simulink model "test_mdl_NI"  (R2018a)
settings: Solver=VariableStepAuto  StartTime=0.0  StopTime=10.0  RelTol=1e-3
(part 5 of 24)

== system test_mdl_NI/CAN_Signal/BCM/PaakRqData1_0x468 ==
  in : Inport
  KeyPadCodeProg_D_Stat : Subsystem
  PaakTrgtData_D_Rq : Subsystem
  PaakTrgtPssvData_No_Rq : Subsystem
  PaakTrgtRollCode_No_Rq : Subsystem
  PaakTrgtType_D_Rq : Subsystem
  PaakTrgtZone_D_Rq : Subsystem
  bus_creator : BusCreator  Inputs=6
  bus_selector : BusSelector  OutputSignals=PaakTrgtPssvData_No_Rq,PaakTrgtData_D_Rq,PaakTrgtRollCode_No_Rq,PaakTrgtType_D_Rq,PaakTrgtZone_D_Rq,KeyPadCodeProg_D_Stat
  out_port : Outport
  wires:
  bus_creator/1 -> out_port/1  "PaakRqData1_0x468"
  PaakTrgtPssvData_No_Rq/1(out) -> bus_creator/1  "PaakTrgtPssvData_No_Rq"
  PaakTrgtData_D_Rq/1(out) -> bus_creator/2  "PaakTrgtData_D_Rq"
  PaakTrgtRollCode_No_Rq/1(out) -> bus_creator/3  "PaakTrgtRollCode_No_Rq"
  PaakTrgtType_D_Rq/1(out) -> bus_creator/4  "PaakTrgtType_D_Rq"
  PaakTrgtZone_D_Rq/1(out) -> bus_creator/5  "PaakTrgtZone_D_Rq"
  KeyPadCodeProg_D_Stat/1(out) -> bus_creator/6  "KeyPadCodeProg_D_Stat"
  bus_selector/1 -> PaakTrgtPssvData_No_Rq/1(in)  "<PaakTrgtPssvData_No_Rq>"
  bus_selector/2 -> PaakTrgtData_D_Rq/1(in)  "<PaakTrgtData_D_Rq>"
  bus_selector/3 -> PaakTrgtRollCode_No_Rq/1(in)  "<PaakTrgtRollCode_No_Rq>"
  bus_selector/4 -> PaakTrgtType_D_Rq/1(in)  "<PaakTrgtType_D_Rq>"
  bus_selector/5 -> PaakTrgtZone_D_Rq/1(in)  "<PaakTrgtZone_D_Rq>"
  bus_selector/6 -> KeyPadCodeProg_D_Stat/1(in)  "<KeyPadCodeProg_D_Stat>"
  in/1 -> bus_selector/1

== system test_mdl_NI/CAN_Signal/BCM/PaakRqData2_0x469 ==
  in : Inport
  PaakTrgtActvData_No_Rq : Subsystem
  bus_creator : BusCreator  Inputs=1
  bus_selector : BusSelector  OutputSignals=PaakTrgtActvData_No_Rq
  out_port : Outport
  wires:
  bus_creator/1 -> out_port/1  "PaakRqData2_0x469"
  PaakTrgtActvData_No_Rq/1(out) -> bus_creator/1  "PaakTrgtActvData_No_Rq"
  bus_selector/1 -> PaakTrgtActvData_No_Rq/1(in)  "<PaakTrgtActvData_No_Rq>"
  in/1 -> bus_selector/1

== system test_mdl_NI/CAN_Signal/BCM/Personality_BCM2_Data_0x3EB ==
  in : Inport
  AssocConfirm_D_Actl : Subsystem
  EmPrflKeyAssoc_D_Stat : Subsystem
  EmPrflNo_D_Stat : Subsystem
  Pers1Key_D_Stat : Subsystem
  Pers2Key_D_Stat : Subsystem
  Pers3Key_D_Stat : Subsystem
  Pers4Key_D_Stat : Subsystem
  PersConflict_D_Actl : Subsystem
  PersNoPos_D_Actl : Subsystem
  PersNo_D_Actl : Subsystem
  PersRecallSrc_D_Actl : Subsystem
  PersSetupAccessCtrl : Subsystem
  PersSetupRestr_D_Actl : Subsystem
  PersSetup_No_Actl : Subsystem
  RecallEvent_No_Cnt : Subsystem
  VehKeyActv_D_Stat : Subsystem
  bus_creator : BusCreator  Inputs=16
  bus_selector : BusSelector  OutputSignals=RecallEvent_No_Cnt,AssocConfirm_D_Actl,Pers1Key_D_Stat,PersNo_D_Actl,PersConflict_D_Actl,PersSetupRestr_D_Actl,PersSetupAccessCtrl,PersNoPos_D_Actl,PersSetup_No_Actl,VehKeyActv_D_Stat,Pers2Key_D_Stat,Pers3Key_D_Stat,EmPrflKeyAssoc_D_Stat,EmPrflNo_D_Stat,Pers4Key_D_Stat,PersRecallSrc_D_Actl
  out_port : Outport
  wires:
  bus_creator/1 -> out_port/1  "Personality_BCM2_Data_0x3EB"
  RecallEvent_No_Cnt/1(out) -> bus_creator/1  "RecallEvent_No_Cnt"
  AssocConfirm_D_Actl/1(out) -> bus_creator/2  "AssocConfirm_D_Actl"
  Pers1Key_D_Stat/1(out) -> bus_creator/3  "Pers1Key_D_Stat"
  PersNo_D_Actl/1(out) -> bus_creator/4  "PersNo_D_Actl"
  PersConflict_D_Actl/1(out) -> bus_creator/5  "PersConflict_D_Actl"
  PersSetupRestr_D_Actl/1(out) -> bus_creator/6  "PersSetupRestr_D_Actl"
  PersSetupAccessCtrl/1(out) -> bus_creator/7  "PersSetupAccessCtrl"
  PersNoPos_D_Actl/1(out) -> bus_creator/8  "PersNoPos_D_Actl"
  PersSetup_No_Actl/1(out) -> bus_creator/9  "PersSetup_No_Actl"
  VehKeyActv_D_Stat/1(out) -> bus_creator/10  "VehKeyActv_D_Stat"
  Pers2Key_D_Stat/1(out) -> bus_creator/11  "Pers2Key_D_Stat"
  Pers3Key_D_Stat/1(out) -> bus_creator/12  "Pers3Key_D_Stat"
  EmPrflKeyAssoc_D_Stat/1(out) -> bus_creator/13  "EmPrflKeyAssoc_D_Stat"
  EmPrflNo_D_Stat/1(out) -> bus_creator/14  "EmPrflNo_D_Stat"
  Pers4Key_D_Stat/1(out) -> bus_creator/15  "Pers4Key_D_Stat"
  PersRecallSrc_D_Actl/1(out) -> bus_creator/16  "PersRecallSrc_D_Actl"
  bus_selector/1 -> RecallEvent_No_Cnt/1(in)  "<RecallEvent_No_Cnt>"
  bus_selector/2 -> AssocConfirm_D_Actl/1(in)  "<AssocConfirm_D_Actl>"
  bus_selector/3 -> Pers1Key_D_Stat/1(in)  "<Pers1Key_D_Stat>"
  bus_selector/4 -> PersNo_D_Actl/1(in)  "<PersNo_D_Actl>"
  bus_selector/5 -> PersConflict_D_Actl/1(in)  "<PersConflict_D_Actl>"
  bus_selector/6 -> PersSetupRestr_D_Actl/1(in)  "<PersSetupRestr_D_Actl>"
  bus_selector/7 -> PersSetupAccessCtrl/1(in)  "<PersSetupAccessCtrl>"
  bus_selector/8 -> PersNoPos_D_Actl/1(in)  "<PersNoPos_D_Actl>"
  bus_selector/9 -> PersSetup_No_Actl/1(in)  "<PersSetup_No_Actl>"
  bus_selector/10 -> VehKeyActv_D_Stat/1(in)  "<VehKeyActv_D_Stat>"
  bus_selector/11 -> Pers2Key_D_Stat/1(in)  "<Pers2Key_D_Stat>"
  bus_selector/12 -> Pers3Key_D_Stat/1(in)  "<Pers3Key_D_Stat>"
  bus_selector/13 -> EmPrflKeyAssoc_D_Stat/1(in)  "<EmPrflKeyAssoc_D_Stat>"
  bus_selector/14 -> EmPrflNo_D_Stat/1(in)  "<EmPrflNo_D_Stat>"
  bus_selector/15 -> Pers4Key_D_Stat/1(in)  "<Pers4Key_D_Stat>"
  bus_selector/16 -> PersRecallSrc_D_Actl/1(in)  "<PersRecallSrc_D_Actl>"
  in/1 -> bus_selector/1

== system test_mdl_NI/CAN_Signal/BCM/Personality_BCM_Data_0x3E3 ==
  in : Inport
  FeatConfigBcmActl : Subsystem
  FeatNoBcm_No_Actl : Subsystem
  FobAssocChime_B_Rq : Subsystem
  LightAmbColor_No_Actl : Subsystem
  LightAmbIntsty_No_Actl : Subsystem
  PersIndexBcm_D_Actl : Subsystem
  bus_creator : BusCreator  Inputs=6
  bus_selector : BusSelector  OutputSignals=FeatConfigBcmActl,FeatNoBcm_No_Actl,PersIndexBcm_D_Actl,FobAssocChime_B_Rq,LightAmbColor_No_Actl,LightAmbIntsty_No_Actl
  out_port : Outport
  wires:
  bus_creator/1 -> out_port/1  "Personality_BCM_Data_0x3E3"
  FeatConfigBcmActl/1(out) -> bus_creator/1  "FeatConfigBcmActl"
  FeatNoBcm_No_Actl/1(out) -> bus_creator/2  "FeatNoBcm_No_Actl"
  PersIndexBcm_D_Actl/1(out) -> bus_creator/3  "PersIndexBcm_D_Actl"
  FobAssocChime_B_Rq/1(out) -> bus_creator/4  "FobAssocChime_B_Rq"
  LightAmbColor_No_Actl/1(out) -> bus_creator/5  "LightAmbColor_No_Actl"
  LightAmbIntsty_No_Actl/1(out) -> bus_creator/6  "LightAmbIntsty_No_Actl"
  bus_selector/1 -> FeatConfigBcmActl/1(in)  "<FeatConfigBcmActl>"
  bus_selector/2 -> FeatNoBcm_No_Actl/1(in)  "<FeatNoBcm_No_Actl>"
  bus_selector/3 -> PersIndexBcm_D_Actl/1(in)  "<PersIndexBcm_D_Actl>"
  bus_selector/4 -> FobAssocChime_B_Rq/1(in)  "<FobAssocChime_B_Rq>"
  bus_selector/5 -> LightAmbColor_No_Actl/1(in)  "<LightAmbColor_No_Actl>"
  bus_selector/6 -> LightAmbIntsty_No_Actl/1(in)  "<LightAmbIntsty_No_Actl>"
  in/1 -> bus_selector/1

== system test_mdl_NI/CAN_Signal/BCM/Power_Stat_0x456 ==
  in : Inport
  RstrnMdulePw_D_Falt : Subsystem
  bus_creator : BusCreator  Inputs=1
  bus_selector : BusSelector  OutputSignals=RstrnMdulePw_D_Falt
  out_port : Outport
  wires:
  bus_creator/1 -> out_port/1  "Power_Stat_0x456"
  RstrnMdulePw_D_Falt/1(out) -> bus_creator/1  "RstrnMdulePw_D_Falt"
  bus_selector/1 -> RstrnMdulePw_D_Falt/1(in)  "<RstrnMdulePw_D_Falt>"
  in/1 -> bus_selector/1

== system test_mdl_NI/CAN_Signal/BCM/RKE_Packet_0x3B6 ==
  in : Inport
  Modulation_Ctrl : Subsystem
  RemoteKey_Info_Ctrl : Subsystem
  RemoteKey_Info_Index : Subsystem
  RemoteKey_Info_MaxInd : Subsystem
  RemoteKey_Info_TIC : Subsystem
  TirePress_Filter_Ctrl : Subsystem
  bus_creator : BusCreator  Inputs=6
  bus_selector : BusSelector  OutputSignals=TirePress_Filter_Ctrl,Modulation_Ctrl,RemoteKey_Info_Ctrl,RemoteKey_Info_Index,RemoteKey_Info_MaxInd,RemoteKey_Info_TIC
  out_port : Outport
  wires:
  bus_creator/1 -> out_port/1  "RKE_Packet_0x3B6"
  TirePress_Filter_Ctrl/1(out) -> bus_creator/1  "TirePress_Filter_Ctrl"
  Modulation_Ctrl/1(out) -> bus_creator/2  "Modulation_Ctrl"
  RemoteKey_Info_Ctrl/1(out) -> bus_creator/3  "RemoteKey_Info_Ctrl"
  RemoteKey_Info_Index/1(out) -> bus_creator/4  "RemoteKey_Info_Index"
  RemoteKey_Info_MaxInd/1(out) -> bus_creator/5  "RemoteKey_Info_MaxInd"
  RemoteKey_Info_TIC/1(out) -> bus_creator/6  "RemoteKey_Info_TIC"
  bus_selector/1 -> TirePress_Filter_Ctrl/1(in)  "<TirePress_Filter_Ctrl>"
  bus_selector/2 -> Modulation_Ctrl/1(in)  "<Modulation_Ctrl>"
  bus_selector/3 -> RemoteKey_Info_Ctrl/1(in)  "<RemoteKey_Info_Ctrl>"
  bus_selector/4 -> RemoteKey_Info_Index/1(in)  "<RemoteKey_Info_Index>"
  bus_selector/5 -> RemoteKey_Info_MaxInd/1(in)  "<RemoteKey_Info_MaxInd>"
  bus_selector/6 -> RemoteKey_Info_TIC/1(in)  "<RemoteKey_Info_TIC>"
  in/1 -> bus_selector/1

== system test_mdl_NI/CAN_Signal/BCM/TPM_Frame_0x3B7 ==
  in : Inport
  TirePress_Info_ID : Subsystem
  TirePress_Info_Index : Subsystem
  TirePress_Info_MaxInd : Subsystem
  bus_creator : BusCreator  Inputs=3
  bus_selector : BusSelector  OutputSignals=TirePress_Info_Index,TirePress_Info_MaxInd,TirePress_Info_ID
  out_port : Outport
  wires:
  bus_creator/1 -> out_port/1  "TPM_Frame_0x3B7"
  TirePress_Info_Index/1(out) -> bus_creator/1  "TirePress_Info_Index"
  TirePress_Info_MaxInd/1(out) -> bus_creator/2  "TirePress_Info_MaxInd"
  TirePress_Info_ID/1(out) -> bus_creator/3  "TirePress_Info_ID"
  bus_selector/1 -> TirePress_Info_Index/1(in)  "<TirePress_Info_Index>"
  bus_selector/2 -> TirePress_Info_MaxInd/1(in)  "<TirePress_Info_MaxInd>"
  bus_selector/3 -> TirePress_Info_ID/1(in)  "<TirePress_Info_ID>"
  in/1 -> bus_selector/1

== system test_mdl_NI/CAN_Signal/BCM/Tire_Pressure_Data_0x3B5 ==
  in : Inport
  Tire_Press_LF_Data : Subsystem
  Tire_Press_LR_OLR_Data : Subsystem
  Tire_Press_RF_Data : Subsystem
  Tire_Press_RR_ORR_Data : Subsystem
  bus_creator : BusCreator  Inputs=4
  bus_selector : BusSelector  OutputSignals=Tire_Press_LF_Data,Tire_Press_RF_Data,Tire_Press_RR_ORR_Data,Tire_Press_LR_OLR_Data
  out_port : Outport
  wires:
  bus_creator/1 -> out_port/1  "Tire_Pressure_Data_0x3B5"
  Tire_Press_LF_Data/1(out) -> bus_creator/1  "Tire_Press_LF_Data"
  Tire_Press_RF_Data/1(out) -> bus_creator/2  "Tire_Press_RF_Data"
  Tire_Press_RR_ORR_Data/1(out) -> bus_creator/3  "Tire_Press_RR_ORR_Data"
  Tire_Press_LR_OLR_Data/1(out) -> bus_creator/4  "Tire_Press_LR_OLR_Data"
  bus_selector/1 -> Tire_Press_LF_Data/1(in)  "<Tire_Press_LF_Data>"
  bus_selector/2 -> Tire_Press_RF_Data/1(in)  "<Tire_Press_RF_Data>"
  bus_selector/3 -> Tire_Press_RR_ORR_Data/1(in)  "<Tire_Press_RR_ORR_Data>"
  bus_selector/4 -> Tire_Press_LR_OLR_Data/1(in)  "<Tire_Press_LR_OLR_Data>"
  in/1 -> bus_selector/1

== system test_mdl_NI/CAN_Signal/BCM/Tire_Pressure_Data_DRW_0x3B8 ==
  in : Inport
  Tire_Press_ILR_Data : Subsystem
  Tire_Press_IRR_Data : Subsystem
  bus_creator : BusCreator  Inputs=2
  bus_selector : BusSelector  OutputSignals=Tire_Press_ILR_Data,Tire_Press_IRR_Data
  out_port : Outport
  wires:
  bus_creator/1 -> out_port/1  "Tire_Pressure_Data_DRW_0x3B8"
  Tire_Press_ILR_Data/1(out) -> bus_creator/1  "Tire_Press_ILR_Data"
  Tire_Press_IRR_Data/1(out) -> bus_creator/2  "Tire_Press_IRR_Data"
  bus_selector/1 -> Tire_Press_ILR_Data/1(in)  "<Tire_Press_ILR_Data>"
  bus_selector/2 -> Tire_Press_IRR_Data/1(in)  "<Tire_Press_IRR_Data>"
  in/1 -> bus_selector/1

== system test_mdl_NI/CAN_Signal/BCM/Tire_Pressure_Stat_0x3B4 ==
  in : Inport
  TirePReset_D_Stat : Subsystem
  Tire_Press_ILR_Stat : Subsystem
  Tire_Press_IRR_Stat : Subsystem
  Tire_Press_LF_Stat : Subsystem
  Tire_Press_LR_OLR_Stat : Subsystem
  Tire_Press_Placrd_Frnt : Subsystem
  Tire_Press_Placrd_Rear : Subsystem
  Tire_Press_RF_Stat : Subsystem
  Tire_Press_RR_ORR_Stat : Subsystem
  Tire_Press_System_Stat : Subsystem
  Tire_Press_Telltale : Subsystem
  bus_creator : BusCreator  Inputs=11
  bus_selector : BusSelector  OutputSignals=Tire_Press_System_Stat,Tire_Press_Telltale,TirePReset_D_Stat,Tire_Press_LF_Stat,Tire_Press_RF_Stat,Tire_Press_RR_ORR_Stat,Tire_Press_LR_OLR_Stat,Tire_Press_IRR_Stat,Tire_Press_ILR_Stat,Tire_Press_Placrd_Frnt,Tire_Press_Placrd_Rear
  out_port : Outport
  wires:
  bus_creator/1 -> out_port/1  "Tire_Pressure_Stat_0x3B4"
  Tire_Press_System_Stat/1(out) -> bus_creator/1  "Tire_Press_System_Stat"
  Tire_Press_Telltale/1(out) -> bus_creator/2  "Tire_Press_Telltale"
  TirePReset_D_Stat/1(out) -> bus_creator/3  "TirePReset_D_Stat"
  Tire_Press_LF_Stat/1(out) -> bus_creator/4  "Tire_Press_LF_Stat"
  Tire_Press_RF_Stat/1(out) -> bus_creator/5  "Tire_Press_RF_Stat"
  Tire_Press_RR_ORR_Stat/1(out) -> bus_creator/6  "Tire_Press_RR_ORR_Stat"
  Tire_Press_LR_OLR_Stat/1(out) -> bus_creator/7  "Tire_Press_LR_OLR_Stat"
  Tire_Press_IRR_Stat/1(out) -> bus_creator/8  "Tire_Press_IRR_Stat"
  Tire_Press_ILR_Stat/1(out) -> bus_creator/9  "Tire_Press_ILR_Stat"
  Tire_Press_Placrd_Frnt/1(out) -> bus_creator/10  "Tire_Press_Placrd_Frnt"
  Tire_Press_Placrd_Rear/1(out) -> bus_creator/11  "Tire_Press_Placrd_Rear"
  bus_selector/1 -> Tire_Press_System_Stat/1(in)  "<Tire_Press_System_Stat>"
  bus_selector/2 -> Tire_Press_Telltale/1(in)  "<Tire_Press_Telltale>"
  bus_selector/3 -> TirePReset_D_Stat/1(in)  "<TirePReset_D_Stat>"
  bus_selector/4 -> Tire_Press_LF_Stat/1(in)  "<Tire_Press_LF_Stat>"
  bus_selector/5 -> Tire_Press_RF_Stat/1(in)  "<Tire_Press_RF_Stat>"
  bus_selector/6 -> Tire_Press_RR_ORR_Stat/1(in)  "<Tire_Press_RR_ORR_Stat>"
  bus_selector/7 -> Tire_Press_LR_OLR_Stat/1(in)  "<Tire_Press_LR_OLR_Stat>"
  bus_selector/8 -> Tire_Press_IRR_Stat/1(in)  "<Tire_Press_IRR_Stat>"
  bus_selector/9 -> Tire_Press_ILR_Stat/1(in)  "<Tire_Press_ILR_Stat>"
  bus_selector/10 -> Tire_Press_Placrd_Frnt/1(in)  "<Tire_Press_Placrd_Frnt>"
  bus_selector/11 -> Tire_Press_Placrd_Rear/1(in)  "<Tire_Press_Placrd_Rear>"
  in/1 -> bus_selector/1

== system test_mdl_NI/CAN_Signal/DSMC/CMR_DSMC_AutoSar_NetwrkMgt ==
  in : Inport
  CMR_DSMC_AutoSarNMControl : Subsystem
  CMR_DSMC_AutoSarNMNodeId : Subsystem
  CMR_DSMC_AutoSarNMReserve2 : Subsystem
  CMR_DSMC_AutoSarNMReserve3 : Subsystem
  CMR_DSMC_AutoSarNMReserve4 : Subsystem
  CMR_DSMC_AutoSarNMReserved : Subsystem
  CMR_DSMC_GWNMProxY : Subsystem
  CMR_DSMC_GWOnBoardTester : Subsystem
  bus_creator : BusCreator  Inputs=8
  bus_selector : BusSelector  OutputSignals=CMR_DSMC_AutoSarNMControl,CMR_DSMC_AutoSarNMNodeId,CMR_DSMC_AutoSarNMReserve2,CMR_DSMC_AutoSarNMReserve3,CMR_DSMC_AutoSarNMReserve4,CMR_DSMC_AutoSarNMReserved,CMR_DSMC_GWNMProxY,CMR_DSMC_GWOnBoardTester
  out_port : Outport
  wires:
  bus_creator/1 -> out_port/1  "CMR_DSMC_AutoSar_NetwrkMgt"
  CMR_DSMC_AutoSarNMControl/1(out) -> bus_creator/1  "CMR_DSMC_AutoSarNMControl"
  CMR_DSMC_AutoSarNMNodeId/1(out) -> bus_creator/2  "CMR_DSMC_AutoSarNMNodeId"
  CMR_DSMC_AutoSarNMReserve2/1(out) -> bus_creator/3  "CMR_DSMC_AutoSarNMReserve2"
  CMR_DSMC_AutoSarNMReserve3/1(out) -> bus_creator/4  "CMR_DSMC_AutoSarNMReserve3"
  CMR_DSMC_AutoSarNMReserve4/1(out) -> bus_creator/5  "CMR_DSMC_AutoSarNMReserve4"
  CMR_DSMC_AutoSarNMReserved/1(out) -> bus_creator/6  "CMR_DSMC_AutoSarNMReserved"
  CMR_DSMC_GWNMProxY/1(out) -> bus_creator/7  "CMR_DSMC_GWNMProxY"
  CMR_DSMC_GWOnBoardTester/1(out) -> bus_creator/8  "CMR_DSMC_GWOnBoardTester"
  bus_selector/1 -> CMR_DSMC_AutoSarNMControl/1(in)  "<CMR_DSMC_AutoSarNMControl>"
  bus_selector/2 -> CMR_DSMC_AutoSarNMNodeId/1(in)  "<CMR_DSMC_AutoSarNMNodeId>"
  bus_selector/3 -> CMR_DSMC_AutoSarNMReserve2/1(in)  "<CMR_DSMC_AutoSarNMReserve2>"
  bus_selector/4 -> CMR_DSMC_AutoSarNMReserve3/1(in)  "<CMR_DSMC_AutoSarNMReserve3>"
  bus_selector/5 -> CMR_DSMC_AutoSarNMReserve4/1(in)  "<CMR_DSMC_AutoSarNMReserve4>"
  bus_selector/6 -> CMR_DSMC_AutoSarNMReserved/1(in)  "<CMR_DSMC_AutoSarNMReserved>"
  bus_selector/7 -> CMR_DSMC_GWNMProxY/1(in)  "<CMR_DSMC_GWNMProxY>"
  bus_selector/8 -> CMR_DSMC_GWOnBoardTester/1(in)  "<CMR_DSMC_GWOnBoardTester>"
  in/1 -> bus_selector/1

== system test_mdl_NI/CAN_Signal/DSMC/DrvStatMonData ==
  in : Inport
  DrvAlertSt_D_Stat : Subsystem
  DrvAttentZone_D_Stat : Subsystem
  DrvCamDrvIR_D_Stat : Subsystem
  DrvCamPassIR_D_Stat : Subsystem
  DrvCamera_D_Stat : Subsystem
  DrvEngLvlConfid_D_Stat : Subsystem
  DrvEngageLevel_D_Stat : Subsystem
  DrvEngageLevel_No_Cnt : Subsystem
  DrvEngageLevel_No_Cs : Subsystem
  DrvImpLvlConfid_D_Stat : Subsystem
  DrvImpairLvl_D_Stat : Subsystem
  bus_creator : BusCreator  Inputs=11
  bus_selector : BusSelector  OutputSignals=DrvAlertSt_D_Stat,DrvAttentZone_D_Stat,DrvCamDrvIR_D_Stat,DrvCamPassIR_D_Stat,DrvCamera_D_Stat,DrvEngLvlConfid_D_Stat,DrvEngageLevel_D_Stat,DrvEngageLevel_No_Cnt,DrvEngageLevel_No_Cs,DrvImpLvlConfid_D_Stat,DrvImpairLvl_D_Stat
  out_port : Outport
  wires:
  bus_creator/1 -> out_port/1  "DrvStatMonData"
  DrvAlertSt_D_Stat/1(out) -> bus_creator/1  "DrvAlertSt_D_Stat"
  DrvAttentZone_D_Stat/1(out) -> bus_creator/2  "DrvAttentZone_D_Stat"
  DrvCamDrvIR_D_Stat/1(out) -> bus_creator/3  "DrvCamDrvIR_D_Stat"
  DrvCamPassIR_D_Stat/1(out) -> bus_creator/4  "DrvCamPassIR_D_Stat"
  DrvCamera_D_Stat/1(out) -> bus_creator/5  "DrvCamera_D_Stat"
  DrvEngLvlConfid_D_Stat/1(out) -> bus_creator/6  "DrvEngLvlConfid_D_Stat"
  DrvEngageLevel_D_Stat/1(out) -> bus_creator/7  "DrvEngageLevel_D_Stat"
  DrvEngageLevel_No_Cnt/1(out) -> bus_creator/8  "DrvEngageLevel_No_Cnt"
  DrvEngageLevel_No_Cs/1(out) -> bus_creator/9  "DrvEngageLevel_No_Cs"
  DrvImpLvlConfid_D_Stat/1(out) -> bus_creator/10  "DrvImpLvlConfid_D_Stat"
  DrvImpairLvl_D_Stat/1(out) -> bus_creator/11  "DrvImpairLvl_D_Stat"
  bus_selector/1 -> DrvAlertSt_D_Stat/1(in)  "<DrvAlertSt_D_Stat>"
  bus_selector/2 -> DrvAttentZone_D_Stat/1(in)  "<DrvAttentZone_D_Stat>"
  bus_selector/3 -> DrvCamDrvIR_D_Stat/1(in)  "<DrvCamDrvIR_D_Stat>"
  bus_selector/4 -> DrvCamPassIR_D_Stat/1(in)  "<DrvCamPassIR_D_Stat>"
  bus_selector/5 -> DrvCamera_D_Stat/1(in)  "<DrvCamera_D_Stat>"
  bus_selector/6 -> DrvEngLvlConfid_D_Stat/1(in)  "<DrvEngLvlConfid_D_Stat>"
  bus_selector/7 -> DrvEngageLevel_D_Stat/1(in)  "<DrvEngageLevel_D_Stat>"
  bus_selector/8 -> DrvEngageLevel_No_Cnt/1(in)  "<DrvEngageLevel_No_Cnt>"
  bus_selector/9 -> DrvEngageLevel_No_Cs/1(in)  "<DrvEngageLevel_No_Cs>"
  bus_selector/10 -> DrvImpLvlConfid_D_Stat/1(in)  "<DrvImpLvlConfid_D_Stat>"
  bus_selector/11 -> DrvImpairLvl_D_Stat/1(in)  "<DrvImpairLvl_D_Stat>"
  in/1 -> bus_selector/1

== system test_mdl_NI/CAN_Signal/DSMC/TesterPhysicalResCMR_DSMC ==
  in : Inport
  TesterPhysicalResCMR_DSMC : Subsystem
  bus_creator : BusCreator  Inputs=1
  bus_selector : BusSelector  OutputSignals=TesterPhysicalResCMR_DSMC
  out_port : Outport
  wires:
  bus_creator/1 -> out_port/1  "TesterPhysicalResCMR_DSMC"
  TesterPhysicalResCMR_DSMC/1(out) -> bus_creator/1  "TesterPhysicalResCMR_DSMC"
  bus_selector/1 -> TesterPhysicalResCMR_DSMC/1(in)  "<TesterPhysicalResCMR_DSMC>"
  in/1 -> bus_selector/1

== system test_mdl_NI/CAN_Signal/ECM_DIESEL PCM PCM_HEV/EngBrakeData_0x165 ==
  in : Inport
  AccEngStat_D_Actl : Subsystem
  AccStopMde_D_Rq : Subsystem
  BPedDrvAppl_D_QF : Subsystem
  BpedDrvAppl_D_Actl : Subsystem
  CcMde_D_Actl : Subsystem
  CcOvrrdActv_B_Actl : Subsystem
  CcStat_D_Actl : Subsystem
  CmbbDeny_B_ActlPrpl : Subsystem
  CmbbEngTqMn_B_Actl : Subsystem
  EngAout_N_MnAllw : Subsystem
  PrplTqMnSat_B_Actl : Subsystem
  Veh_V_DsplyCcSet : Subsystem
  bus_creator : BusCreator  Inputs=12
  bus_selector : BusSelector  OutputSignals=CmbbEngTqMn_B_Actl,CcOvrrdActv_B_Actl,BpedDrvAppl_D_Actl,CmbbDeny_B_ActlPrpl,AccEngStat_D_Actl,BPedDrvAppl_D_QF,CcMde_D_Actl,CcStat_D_Actl,Veh_V_DsplyCcSet,AccStopMde_D_Rq,PrplTqMnSat_B_Actl,EngAout_N_MnAllw
  out_port : Outport
  wires:
  bus_creator/1 -> out_port/1  "EngBrakeData_0x165"
  CmbbEngTqMn_B_Actl/1(out) -> bus_creator/1  "CmbbEngTqMn_B_Actl"
  CcOvrrdActv_B_Actl/1(out) -> bus_creator/2  "CcOvrrdActv_B_Actl"
  BpedDrvAppl_D_Actl/1(out) -> bus_creator/3  "BpedDrvAppl_D_Actl"
  CmbbDeny_B_ActlPrpl/1(out) -> bus_creator/4  "CmbbDeny_B_ActlPrpl"
  AccEngStat_D_Actl/1(out) -> bus_creator/5  "AccEngStat_D_Actl"
  BPedDrvAppl_D_QF/1(out) -> bus_creator/6  "BPedDrvAppl_D_QF"
  CcMde_D_Actl/1(out) -> bus_creator/7  "CcMde_D_Actl"
  CcStat_D_Actl/1(out) -> bus_creator/8  "CcStat_D_Actl"
  Veh_V_DsplyCcSet/1(out) -> bus_creator/9  "Veh_V_DsplyCcSet"
  AccStopMde_D_Rq/1(out) -> bus_creator/10  "AccStopMde_D_Rq"
  PrplTqMnSat_B_Actl/1(out) -> bus_creator/11  "PrplTqMnSat_B_Actl"
  EngAout_N_MnAllw/1(out) -> bus_creator/12  "EngAout_N_MnAllw"
  bus_selector/1 -> CmbbEngTqMn_B_Actl/1(in)  "<CmbbEngTqMn_B_Actl>"
  bus_selector/2 -> CcOvrrdActv_B_Actl/1(in)  "<CcOvrrdActv_B_Actl>"
  bus_selector/3 -> BpedDrvAppl_D_Actl/1(in)  "<BpedDrvAppl_D_Actl>"
  bus_selector/4 -> CmbbDeny_B_ActlPrpl/1(in)  "<CmbbDeny_B_ActlPrpl>"
  bus_selector/5 -> AccEngStat_D_Actl/1(in)  "<AccEngStat_D_Actl>"
  bus_selector/6 -> BPedDrvAppl_D_QF/1(in)  "<BPedDrvAppl_D_QF>"
  bus_selector/7 -> CcMde_D_Actl/1(in)  "<CcMde_D_Actl>"
  bus_selector/8 -> CcStat_D_Actl/1(in)  "<CcStat_D_Actl>"
  bus_selector/9 -> Veh_V_DsplyCcSet/1(in)  "<Veh_V_DsplyCcSet>"
  bus_selector/10 -> AccStopMde_D_Rq/1(in)  "<AccStopMde_D_Rq>"
  bus_selector/11 -> PrplTqMnSat_B_Actl/1(in)  "<PrplTqMnSat_B_Actl>"
  bus_selector/12 -> EngAout_N_MnAllw/1(in)  "<EngAout_N_MnAllw>"
  in/1 -> bus_selector/1

== system test_mdl_NI/CAN_Signal/ECM_DIESEL PCM PCM_HEV/EngVehicleSpThrottle2_0x202 ==
  in : Inport
  GearRvrse_D_Actl : Subsystem
  StrtrMtrCtlMsgTxt_D2_Rq : Subsystem
  StrtrMtrCtlMsgTxt_D_Rq : Subsystem
  StrtrMtrDlyStrt_B_Stat : Subsystem
  VehVActlEng_D_Qf : Subsystem
  VehVActlEng_No_Cnt : Subsystem
  VehVActlEng_No_Cs : Subsystem
  VehVTrlrAid_B_Avail : Subsystem
  Veh_V_ActlEng : Subsystem
  Veh_V_RqCcSet : Subsystem
  bus_creator : BusCreator  Inputs=10
  bus_selector : BusSelector  OutputSignals=StrtrMtrCtlMsgTxt_D_Rq,GearRvrse_D_Actl,StrtrMtrCtlMsgTxt_D2_Rq,VehVActlEng_No_Cs,VehVTrlrAid_B_Avail,VehVActlEng_No_Cnt,StrtrMtrDlyStrt_B_Stat,VehVActlEng_D_Qf,Veh_V_RqCcSet,Veh_V_ActlEng
  out_port : Outport
  wires:
  bus_creator/1 -> out_port/1  "EngVehicleSpThrottle2_0x202"
  StrtrMtrCtlMsgTxt_D_Rq/1(out) -> bus_creator/1  "StrtrMtrCtlMsgTxt_D_Rq"
  GearRvrse_D_Actl/1(out) -> bus_creator/2  "GearRvrse_D_Actl"
  StrtrMtrCtlMsgTxt_D2_Rq/1(out) -> bus_creator/3  "StrtrMtrCtlMsgTxt_D2_Rq"
  VehVActlEng_No_Cs/1(out) -> bus_creator/4  "VehVActlEng_No_Cs"
  VehVTrlrAid_B_Avail/1(out) -> bus_creator/5  "VehVTrlrAid_B_Avail"
  VehVActlEng_No_Cnt/1(out) -> bus_creator/6  "VehVActlEng_No_Cnt"
  StrtrMtrDlyStrt_B_Stat/1(out) -> bus_creator/7  "StrtrMtrDlyStrt_B_Stat"
  VehVActlEng_D_Qf/1(out) -> bus_creator/8  "VehVActlEng_D_Qf"
  Veh_V_RqCcSet/1(out) -> bus_creator/9  "Veh_V_RqCcSet"
  Veh_V_ActlEng/1(out) -> bus_creator/10  "Veh_V_ActlEng"
  bus_selector/1 -> StrtrMtrCtlMsgTxt_D_Rq/1(in)  "<StrtrMtrCtlMsgTxt_D_Rq>"
  bus_selector/2 -> GearRvrse_D_Actl/1(in)  "<GearRvrse_D_Actl>"
  bus_selector/3 -> StrtrMtrCtlMsgTxt_D2_Rq/1(in)  "<StrtrMtrCtlMsgTxt_D2_Rq>"
  bus_selector/4 -> VehVActlEng_No_Cs/1(in)  "<VehVActlEng_No_Cs>"
  bus_selector/5 -> VehVTrlrAid_B_Avail/1(in)  "<VehVTrlrAid_B_Avail>"
  bus_selector/6 -> VehVActlEng_No_Cnt/1(in)  "<VehVActlEng_No_Cnt>"
  bus_selector/7 -> StrtrMtrDlyStrt_B_Stat/1(in)  "<StrtrMtrDlyStrt_B_Stat>"
  bus_selector/8 -> VehVActlEng_D_Qf/1(in)  "<VehVActlEng_D_Qf>"
  bus_selector/9 -> Veh_V_RqCcSet/1(in)  "<Veh_V_RqCcSet>"
  bus_selector/10 -> Veh_V_ActlEng/1(in)  "<Veh_V_ActlEng>"
  in/1 -> bus_selector/1

== system test_mdl_NI/CAN_Signal/ECM_DIESEL PCM PCM_HEV/EngVehicleSpThrottle_0x204 ==
  in : Inport
  ApedPosPcActl_D_Qf : Subsystem
  ApedPosPcActl_No_Cnt : Subsystem
  ApedPosPcActl_No_Cs : Subsystem
  ApedPos_PcRate_ActlArb : Subsystem
  ApedPos_Pc_ActlArb : Subsystem
  EngAout3_N_Actl : Subsystem
  EngAoutNActl_D_QF : Subsystem
  EngAout_N_Actl : Subsystem
  bus_creator : BusCreator  Inputs=8
  bus_selector : BusSelector  OutputSignals=ApedPosPcActl_D_Qf,ApedPosPcActl_No_Cnt,ApedPos_Pc_ActlArb,ApedPos_PcRate_ActlArb,EngAoutNActl_D_QF,EngAout_N_Actl,ApedPosPcActl_No_Cs,EngAout3_N_Actl
  out_port : Outport
  wires:
  bus_creator/1 -> out_port/1  "EngVehicleSpThrottle_0x204"
  ApedPosPcActl_D_Qf/1(out) -> bus_creator/1  "ApedPosPcActl_D_Qf"
  ApedPosPcActl_No_Cnt/1(out) -> bus_creator/2  "ApedPosPcActl_No_Cnt"
  ApedPos_Pc_ActlArb/1(out) -> bus_creator/3  "ApedPos_Pc_ActlArb"
  ApedPos_PcRate_ActlArb/1(out) -> bus_creator/4  "ApedPos_PcRate_ActlArb"
  EngAoutNActl_D_QF/1(out) -> bus_creator/5  "EngAoutNActl_D_QF"
  EngAout_N_Actl/1(out) -> bus_creator/6  "EngAout_N_Actl"
  ApedPosPcActl_No_Cs/1(out) -> bus_creator/7  "ApedPosPcActl_No_Cs"
  EngAout3_N_Actl/1(out) -> bus_creator/8  "EngAout3_N_Actl"
  bus_selector/1 -> ApedPosPcActl_D_Qf/1(in)  "<ApedPosPcActl_D_Qf>"
  bus_selector/2 -> ApedPosPcActl_No_Cnt/1(in)  "<ApedPosPcActl_No_Cnt>"
  bus_selector/3 -> ApedPos_Pc_ActlArb/1(in)  "<ApedPos_Pc_ActlArb>"
  bus_selector/4 -> ApedPos_PcRate_ActlArb/1(in)  "<ApedPos_PcRate_ActlArb>"
  bus_selector/5 -> EngAoutNActl_D_QF/1(in)  "<EngAoutNActl_D_QF>"
  bus_selector/6 -> EngAout_N_Actl/1(in)  "<EngAout_N_Actl>"
  bus_selector/7 -> ApedPosPcActl_No_Cs/1(in)  "<ApedPosPcActl_No_Cs>"
  bus_selector/8 -> EngAout3_N_Actl/1(in)  "<EngAout3_N_Actl>"
  in/1 -> bus_selector/1

== system test_mdl_NI/CAN_Signal/ECM_DIESEL PCM PCM_HEV/EngineClimateData_0x178 ==
  in : Inport
  AirAmbTe_D_Qf : Subsystem
  AirAmb_P_Actl : Subsystem
  AirAmb_Te_Actl : Subsystem
  AirAmb_Te_ActlFilt : Subsystem
  AslChime_B_Rq : Subsystem
  AslIconDsply_D_Rq : Subsystem
  DynoMde_B_Cmd : Subsystem
  EcssLamp_D_RqDsply : Subsystem
  EngAout_Aa_Actl : Subsystem
  GasPrtc_D_RqDsply : Subsystem
  HvacHtrCore2_Te_Actl : Subsystem
  bus_creator : BusCreator  Inputs=11
  bus_selector : BusSelector  OutputSignals=DynoMde_B_Cmd,AslIconDsply_D_Rq,HvacHtrCore2_Te_Actl,GasPrtc_D_RqDsply,EcssLamp_D_RqDsply,EngAout_Aa_Actl,AslChime_B_Rq,AirAmbTe_D_Qf,AirAmb_Te_Actl,AirAmb_P_Actl,AirAmb_Te_ActlFilt
  out_port : Outport
  wires:
  bus_creator/1 -> out_port/1  "EngineClimateData_0x178"
  DynoMde_B_Cmd/1(out) -> bus_creator/1  "DynoMde_B_Cmd"
  AslIconDsply_D_Rq/1(out) -> bus_creator/2  "AslIconDsply_D_Rq"
  HvacHtrCore2_Te_Actl/1(out) -> bus_creator/3  "HvacHtrCore2_Te_Actl"
  GasPrtc_D_RqDsply/1(out) -> bus_creator/4  "GasPrtc_D_RqDsply"
  EcssLamp_D_RqDsply/1(out) -> bus_creator/5  "EcssLamp_D_RqDsply"
  EngAout_Aa_Actl/1(out) -> bus_creator/6  "EngAout_Aa_Actl"
  AslChime_B_Rq/1(out) -> bus_creator/7  "AslChime_B_Rq"
  AirAmbTe_D_Qf/1(out) -> bus_creator/8  "AirAmbTe_D_Qf"
  AirAmb_Te_Actl/1(out) -> bus_creator/9  "AirAmb_Te_Actl"
  AirAmb_P_Actl/1(out) -> bus_creator/10  "AirAmb_P_Actl"
  AirAmb_Te_ActlFilt/1(out) -> bus_creator/11  "AirAmb_Te_ActlFilt"
  bus_selector/1 -> DynoMde_B_Cmd/1(in)  "<DynoMde_B_Cmd>"
  bus_selector/2 -> AslIconDsply_D_Rq/1(in)  "<AslIconDsply_D_Rq>"
  bus_selector/3 -> HvacHtrCore2_Te_Actl/1(in)  "<HvacHtrCore2_Te_Actl>"
  bus_selector/4 -> GasPrtc_D_RqDsply/1(in)  "<GasPrtc_D_RqDsply>"
  bus_selector/5 -> EcssLamp_D_RqDsply/1(in)  "<EcssLamp_D_RqDsply>"
  bus_selector/6 -> EngAout_Aa_Actl/1(in)  "<EngAout_Aa_Actl>"
  bus_selector/7 -> AslChime_B_Rq/1(in)  "<AslChime_B_Rq>"
  bus_selector/8 -> AirAmbTe_D_Qf/1(in)  "<AirAmbTe_D_Qf>"
  bus_selector/9 -> AirAmb_Te_Actl/1(in)  "<AirAmb_Te_Actl>"
  bus_selector/10 -> AirAmb_P_Actl/1(in)  "<AirAmb_P_Actl>"
  bus_selector/11 -> AirAmb_Te_ActlFilt/1(in)  "<AirAmb_Te_ActlFilt>"
  in/1 -> bus_selector/1

== system test_mdl_NI/CAN_Signal/ECM_DIESEL PCM PCM_HEV/EngineData_6_0x156 ==
  in : Inport
  EngClntTe_D_Qf : Subsystem
  EngClnt_Te_Actl : Subsystem
  EngGoutLss_Tq_Est : Subsystem
  EngOil_Te_Actl : Subsystem
  EngOvrhtMitgActv_D_Ind : Subsystem
  bus_creator : BusCreator  Inputs=5
  bus_selector : BusSelector  OutputSignals=EngClnt_Te_Actl,EngOil_Te_Actl,EngGoutLss_Tq_Est,EngOvrhtMitgActv_D_Ind,EngClntTe_D_Qf
  out_port : Outport
  wires:
  bus_creator/1 -> out_port/1  "EngineData_6_0x156"
  EngClnt_Te_Actl/1(out) -> bus_creator/1  "EngClnt_Te_Actl"
  EngOil_Te_Actl/1(out) -> bus_creator/2  "EngOil_Te_Actl"
  EngGoutLss_Tq_Est/1(out) -> bus_creator/3  "EngGoutLss_Tq_Est"
  EngOvrhtMitgActv_D_Ind/1(out) -> bus_creator/4  "EngOvrhtMitgActv_D_Ind"
  EngClntTe_D_Qf/1(out) -> bus_creator/5  "EngClntTe_D_Qf"
  bus_selector/1 -> EngClnt_Te_Actl/1(in)  "<EngClnt_Te_Actl>"
  bus_selector/2 -> EngOil_Te_Actl/1(in)  "<EngOil_Te_Actl>"
  bus_selector/3 -> EngGoutLss_Tq_Est/1(in)  "<EngGoutLss_Tq_Est>"
  bus_selector/4 -> EngOvrhtMitgActv_D_Ind/1(in)  "<EngOvrhtMitgActv_D_Ind>"
  bus_selector/5 -> EngClntTe_D_Qf/1(in)  "<EngClntTe_D_Qf>"
  in/1 -> bus_selector/1

== system test_mdl_NI/CAN_Signal/ECM_DIESEL PCM PCM_HEV/EngineData_7_0x179 ==
  in : Inport
  AirCondClutch_B_Stats : Subsystem
  AirCondRec_B_Rq : Subsystem
  EngOilLife_Pc_Actl : Subsystem
  EngSrvcRqd_B_Rq : Subsystem
  FuelFillInlet_B_Dsply : Subsystem
  FuelFilterLamp_B_Dsply : Subsystem
  FuelFlw_Vl_Dsply : Subsystem
  HvacAirFullOut_B_Rq : Subsystem
  OdoCount : Subsystem
  TrnKickDown_B_RqDrv : Subsystem
  TrnManShifGear_D_IndDrv : Subsystem
  TrnManShif_D_IndDrv : Subsystem
  bus_creator : BusCreator  Inputs=12
  bus_selector : BusSelector  OutputSignals=TrnManShif_D_IndDrv,HvacAirFullOut_B_Rq,TrnKickDown_B_RqDrv,EngSrvcRqd_B_Rq,EngOilLife_Pc_Actl,FuelFillInlet_B_Dsply,OdoCount,AirCondRec_B_Rq,TrnManShifGear_D_IndDrv,AirCondClutch_B_Stats,FuelFilterLamp_B_Dsply,FuelFlw_Vl_Dsply
  out_port : Outport
  wires:
  bus_creator/1 -> out_port/1  "EngineData_7_0x179"
  TrnManShif_D_IndDrv/1(out) -> bus_creator/1  "TrnManShif_D_IndDrv"
  HvacAirFullOut_B_Rq/1(out) -> bus_creator/2  "HvacAirFullOut_B_Rq"
  TrnKickDown_B_RqDrv/1(out) -> bus_creator/3  "TrnKickDown_B_RqDrv"
  EngSrvcRqd_B_Rq/1(out) -> bus_creator/4  "EngSrvcRqd_B_Rq"
  EngOilLife_Pc_Actl/1(out) -> bus_creator/5  "EngOilLife_Pc_Actl"
  FuelFillInlet_B_Dsply/1(out) -> bus_creator/6  "FuelFillInlet_B_Dsply"
  OdoCount/1(out) -> bus_creator/7  "OdoCount"
  AirCondRec_B_Rq/1(out) -> bus_creator/8  "AirCondRec_B_Rq"
  TrnManShifGear_D_IndDrv/1(out) -> bus_creator/9  "TrnManShifGear_D_IndDrv"
  AirCondClutch_B_Stats/1(out) -> bus_creator/10  "AirCondClutch_B_Stats"
  FuelFilterLamp_B_Dsply/1(out) -> bus_creator/11  "FuelFilterLamp_B_Dsply"
  FuelFlw_Vl_Dsply/1(out) -> bus_creator/12  "FuelFlw_Vl_Dsply"
  bus_selector/1 -> TrnManShif_D_IndDrv/1(in)  "<TrnManShif_D_IndDrv>"
  bus_selector/2 -> HvacAirFullOut_B_Rq/1(in)  "<HvacAirFullOut_B_Rq>"
  bus_selector/3 -> TrnKickDown_B_RqDrv/1(in)  "<TrnKickDown_B_RqDrv>"
  bus_selector/4 -> EngSrvcRqd_B_Rq/1(in)  "<EngSrvcRqd_B_Rq>"
  bus_selector/5 -> EngOilLife_Pc_Actl/1(in)  "<EngOilLife_Pc_Actl>"
  bus_selector/6 -> FuelFillInlet_B_Dsply/1(in)  "<FuelFillInlet_B_Dsply>"
  bus_selector/7 -> OdoCount/1(in)  "<OdoCount>"
  bus_selector/8 -> AirCondRec_B_Rq/1(in)  "<AirCondRec_B_Rq>"
  bus_selector/9 -> TrnManShifGear_D_IndDrv/1(in)  "<TrnManShifGear_D_IndDrv>"
  bus_selector/10 -> AirCondClutch_B_Stats/1(in)  "<AirCondClutch_B_Stats>"
  bus_selector/11 -> FuelFilterLamp_B_Dsply/1(in)  "<FuelFilterLamp_B_Dsply>"
  bus_selector/12 -> FuelFlw_Vl_Dsply/1(in)  "<FuelFlw_Vl_Dsply>"
  in/1 -> bus_selector/1

== system test_mdl_NI/CAN_Signal/ECM_DIESEL PCM PCM_HEV/Engine_Clutch_Data_0x42F ==
  in : Inport
  CluPdlPosPcMeas_D_Qf : Subsystem
  CluPdlPos_Pc_Meas : Subsystem
  CluPdl_PcRate_Actl : Subsystem
  EngAoutIdl_N_Ntrl : Subsystem
  EngAout_N_Dsply : Subsystem
  bus_creator : BusCreator  Inputs=5
  bus_selector : BusSelector  OutputSignals=CluPdl_PcRate_Actl,CluPdlPosPcMeas_D_Qf,CluPdlPos_Pc_Meas,EngAoutIdl_N_Ntrl,EngAout_N_Dsply
  out_port : Outport
  wires:
  bus_creator/1 -> out_port/1  "Engine_Clutch_Data_0x42F"
  CluPdl_PcRate_Actl/1(out) -> bus_creator/1  "CluPdl_PcRate_Actl"
  CluPdlPosPcMeas_D_Qf/1(out) -> bus_creator/2  "CluPdlPosPcMeas_D_Qf"
  CluPdlPos_Pc_Meas/1(out) -> bus_creator/3  "CluPdlPos_Pc_Meas"
  EngAoutIdl_N_Ntrl/1(out) -> bus_creator/4  "EngAoutIdl_N_Ntrl"
  EngAout_N_Dsply/1(out) -> bus_creator/5  "EngAout_N_Dsply"
  bus_selector/1 -> CluPdl_PcRate_Actl/1(in)  "<CluPdl_PcRate_Actl>"
  bus_selector/2 -> CluPdlPosPcMeas_D_Qf/1(in)  "<CluPdlPosPcMeas_D_Qf>"
  bus_selector/3 -> CluPdlPos_Pc_Meas/1(in)  "<CluPdlPos_Pc_Meas>"
  bus_selector/4 -> EngAoutIdl_N_Ntrl/1(in)  "<EngAoutIdl_N_Ntrl>"
  bus_selector/5 -> EngAout_N_Dsply/1(in)  "<EngAout_N_Dsply>"
  in/1 -> bus_selector/1

== system test_mdl_NI/CAN_Signal/ECM_DIESEL PCM PCM_HEV/Gear_Shift_by_Wire_3 ==
  in : Inport
  GearSelLck_D_Rq : Subsystem
  PrkBrkActv_D_RqTrnGear : Subsystem
  TrnCmdCnt_B_Actl : Subsystem
  TrnCmdState_B_Actl : Subsystem
  TrnDtpCmd_D_Actl : Subsystem
  TrnGearCmd_No_Cnt : Subsystem
  TrnGearCmd_No_Cs : Subsystem
  TrnGearCmd_Pc_ActlPt : Subsystem
  TrnGearMsgTxt_D_Rq : Subsystem
  TrnGearNtmAllow_B_Stat : Subsystem
  TrnGear_D_RqPt : Subsystem
  TrnLvrV_D_Rq : Subsystem
  TrnNtrlTowCmd_D_Actl : Subsystem
  TrnSbwSysHlth_D_Actl : Subsystem
  TrnValidGear_D_Cnfm : Subsystem
  bus_creator : BusCreator  Inputs=15
  bus_selector : BusSelector  OutputSignals=GearSelLck_D_Rq,PrkBrkActv_D_RqTrnGear,TrnCmdCnt_B_Actl,TrnCmdState_B_Actl,TrnDtpCmd_D_Actl,TrnGearCmd_No_Cnt,TrnGearCmd_No_Cs,TrnGearCmd_Pc_ActlPt,TrnGearMsgTxt_D_Rq,TrnGearNtmAllow_B_Stat,TrnGear_D_RqPt,TrnLvrV_D_Rq,TrnNtrlTowCmd_D_Actl,TrnSbwSysHlth_D_Actl,TrnValidGear_D_Cnfm
  out_port : Outport
  wires:
  bus_creator/1 -> out_port/1  "Gear_Shift_by_Wire_3"
  GearSelLck_D_Rq/1(out) -> bus_creator/1  "GearSelLck_D_Rq"
  PrkBrkActv_D_RqTrnGear/1(out) -> bus_creator/2  "PrkBrkActv_D_RqTrnGear"
  TrnCmdCnt_B_Actl/1(out) -> bus_creator/3  "TrnCmdCnt_B_Actl"
  TrnCmdState_B_Actl/1(out) -> bus_creator/4  "TrnCmdState_B_Actl"
  TrnDtpCmd_D_Actl/1(out) -> bus_creator/5  "TrnDtpCmd_D_Actl"
  TrnGearCmd_No_Cnt/1(out) -> bus_creator/6  "TrnGearCmd_No_Cnt"
  TrnGearCmd_No_Cs/1(out) -> bus_creator/7  "TrnGearCmd_No_Cs"
  TrnGearCmd_Pc_ActlPt/1(out) -> bus_creator/8  "TrnGearCmd_Pc_ActlPt"
  TrnGearMsgTxt_D_Rq/1(out) -> bus_creator/9  "TrnGearMsgTxt_D_Rq"
  TrnGearNtmAllow_B_Stat/1(out) -> bus_creator/10  "TrnGearNtmAllow_B_Stat"
  TrnGear_D_RqPt/1(out) -> bus_creator/11  "TrnGear_D_RqPt"
  TrnLvrV_D_Rq/1(out) -> bus_creator/12  "TrnLvrV_D_Rq"
  TrnNtrlTowCmd_D_Actl/1(out) -> bus_creator/13  "TrnNtrlTowCmd_D_Actl"
  TrnSbwSysHlth_D_Actl/1(out) -> bus_creator/14  "TrnSbwSysHlth_D_Actl"
  TrnValidGear_D_Cnfm/1(out) -> bus_creator/15  "TrnValidGear_D_Cnfm"
  bus_selector/1 -> GearSelLck_D_Rq/1(in)  "<GearSelLck_D_Rq>"
  bus_selector/2 -> PrkBrkActv_D_RqTrnGear/1(in)  "<PrkBrkActv_D_RqTrnGear>"
  bus_selector/3 -> TrnCmdCnt_B_Actl/1(in)  "<TrnCmdCnt_B_Actl>"
  bus_selector/4 -> TrnCmdState_B_Actl/1(in)  "<TrnCmdState_B_Actl>"
  bus_selector/5 -> TrnDtpCmd_D_Actl/1(in)  "<TrnDtpCmd_D_Actl>"
  bus_selector/6 -> TrnGearCmd_No_Cnt/1(in)  "<TrnGearCmd_No_Cnt>"
  bus_selector/7 -> TrnGearCmd_No_Cs/1(in)  "<TrnGearCmd_No_Cs>"
  bus_selector/8 -> TrnGearCmd_Pc_ActlPt/1(in)  "<TrnGearCmd_Pc_ActlPt>"
  bus_selector/9 -> TrnGearMsgTxt_D_Rq/1(in)  "<TrnGearMsgTxt_D_Rq>"
  bus_selector/10 -> TrnGearNtmAllow_B_Stat/1(in)  "<TrnGearNtmAllow_B_Stat>"
  bus_selector/11 -> TrnGear_D_RqPt/1(in)  "<TrnGear_D_RqPt>"
  bus_selector/12 -> TrnLvrV_D_Rq/1(in)  "<TrnLvrV_D_Rq>"
  bus_selector/13 -> TrnNtrlTowCmd_D_Actl/1(in)  "<TrnNtrlTowCmd_D_Actl>"
  bus_selector/14 -> TrnSbwSysHlth_D_Actl/1(in)  "<TrnSbwSysHlth_D_Actl>"
  bus_selector/15 -> TrnValidGear_D_Cnfm/1(in)  "<TrnValidGear_D_Cnfm>"
  in/1 -> bus_selector/1

== system test_mdl_NI/CAN_Signal/ECM_DIESEL PCM PCM_HEV/Global_PATS_TargetInfo_0x47 ==
  in : Inport
  bus_creator : BusCreator  Inputs=3
  bus_selector : BusSelector  OutputSignals=immoTarget1Status,immoTarget1Cmd,immoTarget1Data
  immoTarget1Cmd : Subsystem
  immoTarget1Data : Subsystem
  immoTarget1Status : Subsystem
  out_port : Outport
  wires:
  bus_creator/1 -> out_port/1  "Global_PATS_TargetInfo_0x47"
  immoTarget1Status/1(out) -> bus_creator/1  "immoTarget1Status"
  immoTarget1Cmd/1(out) -> bus_creator/2  "immoTarget1Cmd"
  immoTarget1Data/1(out) -> bus_creator/3  "immoTarget1Data"
  bus_selector/1 -> immoTarget1Status/1(in)  "<immoTarget1Status>"
  bus_selector/2 -> immoTarget1Cmd/1(in)  "<immoTarget1Cmd>"
  bus_selector/3 -> immoTarget1Data/1(in)  "<immoTarget1Data>"
  in/1 -> bus_selector/1

== system test_mdl_NI/CAN_Signal/ECM_DIESEL PCM PCM_HEV/HEV_Powertrain_Data2 ==
  in : Inport
  BattTracCnnct_D_Rq : Subsystem
  PrplTqMnRgen_B_Actl : Subsystem
  WhlDirAvgDrv_D_Actl : Subsystem
  bus_creator : BusCreator  Inputs=3
  bus_selector : BusSelector  OutputSignals=BattTracCnnct_D_Rq,PrplTqMnRgen_B_Actl,WhlDirAvgDrv_D_Actl
  out_port : Outport
  wires:
  bus_creator/1 -> out_port/1  "HEV_Powertrain_Data2"
  BattTracCnnct_D_Rq/1(out) -> bus_creator/1  "BattTracCnnct_D_Rq"
  PrplTqMnRgen_B_Actl/1(out) -> bus_creator/2  "PrplTqMnRgen_B_Actl"
  WhlDirAvgDrv_D_Actl/1(out) -> bus_creator/3  "WhlDirAvgDrv_D_Actl"
  bus_selector/1 -> BattTracCnnct_D_Rq/1(in)  "<BattTracCnnct_D_Rq>"
  bus_selector/2 -> PrplTqMnRgen_B_Actl/1(in)  "<PrplTqMnRgen_B_Actl>"
  bus_selector/3 -> WhlDirAvgDrv_D_Actl/1(in)  "<WhlDirAvgDrv_D_Actl>"
  in/1 -> bus_selector/1

== system test_mdl_NI/CAN_Signal/ECM_DIESEL PCM PCM_HEV/PCM_AutoSar_NetworkMgmt_0x595 ==
  in : Inport
  PCM_AutoSarNMControl : Subsystem
  PCM_AutoSarNMNodeId : Subsystem
  PCM_AutoSarNMReserved1 : Subsystem
  PCM_AutoSarNMReserved2 : Subsystem
  PCM_AutoSarNMReserved3 : Subsystem
  PCM_AutoSarNMReserved4 : Subsystem
  PCM_GWNMProxy : Subsystem
  PCM_GWOnBoardTester : Subsystem
  bus_creator : BusCreator  Inputs=8
  bus_selector : BusSelector  OutputSignals=PCM_AutoSarNMNodeId,PCM_AutoSarNMControl,PCM_AutoSarNMReserved1,PCM_AutoSarNMReserved2,PCM_GWOnBoardTester,PCM_GWNMProxy,PCM_AutoSarNMReserved3,PCM_AutoSarNMReserved4
  out_port : Outport
  wires:
  bus_creator/1 -> out_port/1  "PCM_AutoSar_NetworkMgmt_0x595"
  PCM_AutoSarNMNodeId/1(out) -> bus_creator/1  "PCM_AutoSarNMNodeId"
  PCM_AutoSarNMControl/1(out) -> bus_creator/2  "PCM_AutoSarNMControl"
  PCM_AutoSarNMReserved1/1(out) -> bus_creator/3  "PCM_AutoSarNMReserved1"
  PCM_AutoSarNMReserved2/1(out) -> bus_creator/4  "PCM_AutoSarNMReserved2"
  PCM_GWOnBoardTester/1(out) -> bus_creator/5  "PCM_GWOnBoardTester"
  PCM_GWNMProxy/1(out) -> bus_creator/6  "PCM_GWNMProxy"
  PCM_AutoSarNMReserved3/1(out) -> bus_creator/7  "PCM_AutoSarNMReserved3"
  PCM_AutoSarNMReserved4/1(out) -> bus_creator/8  "PCM_AutoSarNMReserved4"
  bus_selector/1 -> PCM_AutoSarNMNodeId/1(in)  "<PCM_AutoSarNMNodeId>"
  bus_selector/2 -> PCM_AutoSarNMControl/1(in)  "<PCM_AutoSarNMControl>"
  bus_selector/3 -> PCM_AutoSarNMReserved1/1(in)  "<PCM_AutoSarNMReserved1>"
  bus_selector/4 -> PCM_AutoSarNMReserved2/1(in)  "<PCM_AutoSarNMReserved2>"
  bus_selector/5 -> PCM_GWOnBoardTester/1(in)  "<PCM_GWOnBoardTester>"
  bus_selector/6 -> PCM_GWNMProxy/1(in)  "<PCM_GWNMProxy>"
  bus_selector/7 -> PCM_AutoSarNMReserved3/1(in)  "<PCM_AutoSarNMReserved3>"
  bus_selector/8 -> PCM_AutoSarNMReserved4/1(in)  "<PCM_AutoSarNMReserved4>"
  in/1 -> bus_selector/1

== system test_mdl_NI/CAN_Signal/ECM_DIESEL PCM PCM_HEV/PCM_Rapid_Data_Response_1_0x6A0 ==
  in : Inport
  UUDTPCMResponse1 : Subsystem
  bus_creator : BusCreator  Inputs=1
  bus_selector : BusSelector  OutputSignals=UUDTPCMResponse1
  out_port : Outport
  wires:
  bus_creator/1 -> out_port/1  "PCM_Rapid_Data_Response_1_0x6A0"
  UUDTPCMResponse1/1(out) -> bus_creator/1  "UUDTPCMResponse1"
  bus_selector/1 -> UUDTPCMResponse1/1(in)  "<UUDTPCMResponse1>"
  in/1 -> bus_selector/1

== system test_mdl_NI/CAN_Signal/ECM_DIESEL PCM PCM_HEV/PowertrainData_10 ==
  in : Inport
  GearEngag_D_Actl : Subsystem
  GearLvr_D_ActlDrv : Subsystem
  GearPos_D_Actl : Subsystem
  GearPos_D_Trg : Subsystem
  GearPos_No_Cnt : Subsystem
  GearPos_No_Cs : Subsystem
  TrnIgnOffDly_T_Rq : Subsystem
  TrnPrkSys_D_Actl : Subsystem
  TrnRng_D_Rq : Subsystem
  bus_creator : BusCreator  Inputs=9
  bus_selector : BusSelector  OutputSignals=GearEngag_D_Actl,GearLvr_D_ActlDrv,GearPos_D_Actl,GearPos_D_Trg,GearPos_No_Cnt,GearPos_No_Cs,TrnIgnOffDly_T_Rq,TrnPrkSys_D_Actl,TrnRng_D_Rq
  out_port : Outport
  wires:
  bus_creator/1 -> out_port/1  "PowertrainData_10"
  GearEngag_D_Actl/1(out) -> bus_creator/1  "GearEngag_D_Actl"
  GearLvr_D_ActlDrv/1(out) -> bus_creator/2  "GearLvr_D_ActlDrv"
  GearPos_D_Actl/1(out) -> bus_creator/3  "GearPos_D_Actl"
  GearPos_D_Trg/1(out) -> bus_creator/4  "GearPos_D_Trg"
  GearPos_No_Cnt/1(out) -> bus_creator/5  "GearPos_No_Cnt"
  GearPos_No_Cs/1(out) -> bus_creator/6  "GearPos_No_Cs"
  TrnIgnOffDly_T_Rq/1(out) -> bus_creator/7  "TrnIgnOffDly_T_Rq"
  TrnPrkSys_D_Actl/1(out) -> bus_creator/8  "TrnPrkSys_D_Actl"
  TrnRng_D_Rq/1(out) -> bus_creator/9  "TrnRng_D_Rq"
  bus_selector/1 -> GearEngag_D_Actl/1(in)  "<GearEngag_D_Actl>"
  bus_selector/2 -> GearLvr_D_ActlDrv/1(in)  "<GearLvr_D_ActlDrv>"
  bus_selector/3 -> GearPos_D_Actl/1(in)  "<GearPos_D_Actl>"
  bus_selector/4 -> GearPos_D_Trg/1(in)  "<GearPos_D_Trg>"
  bus_selector/5 -> GearPos_No_Cnt/1(in)  "<GearPos_No_Cnt>"
  bus_selector/6 -> GearPos_No_Cs/1(in)  "<GearPos_No_Cs>"
  bus_selector/7 -> TrnIgnOffDly_T_Rq/1(in)  "<TrnIgnOffDly_T_Rq>"
  bus_selector/8 -> TrnPrkSys_D_Actl/1(in)  "<TrnPrkSys_D_Actl>"
  bus_selector/9 -> TrnRng_D_Rq/1(in)  "<TrnRng_D_Rq>"
  in/1 -> bus_selector/1

== system test_mdl_NI/CAN_Signal/ECM_DIESEL PCM PCM_HEV/PowertrainData_1_0x421 ==
  in : Inport
  AirCondFluidHi_P_Actl : Subsystem
  CoolantFanStepAct : Subsystem
  ECMMILRequest : Subsystem
  EngIdlShutDown_D_Stat : Subsystem
  EngIdlShutDwnTxt_D_Rq : Subsystem
  FUEL_ALCOHOL_PERCNT : Subsystem
  FohEng_D_Rq : Subsystem
  OilPressureWarning : Subsystem
  TrnTotLss_Tq_Est : Subsystem
  TrnTotTq_Rt_Est : Subsystem
  VehVLimActv_B_Actl : Subsystem
  VehVLimStat_D_Actl : Subsystem
  bus_creator : BusCreator  Inputs=12
  bus_selector : BusSelector  OutputSignals=VehVLimActv_B_Actl,VehVLimStat_D_Actl,ECMMILRequest,FohEng_D_Rq,EngIdlShutDown_D_Stat,CoolantFanStepAct,OilPressureWarning,EngIdlShutDwnTxt_D_Rq,TrnTotLss_Tq_Est,TrnTotTq_Rt_Est,AirCondFluidHi_P_Actl,FUEL_ALCOHOL_PERCNT
  out_port : Outport
  wires:
  bus_creator/1 -> out_port/1  "PowertrainData_1_0x421"
  VehVLimActv_B_Actl/1(out) -> bus_creator/1  "VehVLimActv_B_Actl"
  VehVLimStat_D_Actl/1(out) -> bus_creator/2  "VehVLimStat_D_Actl"
  ECMMILRequest/1(out) -> bus_creator/3  "ECMMILRequest"
  FohEng_D_Rq/1(out) -> bus_creator/4  "FohEng_D_Rq"
  EngIdlShutDown_D_Stat/1(out) -> bus_creator/5  "EngIdlShutDown_D_Stat"
  CoolantFanStepAct/1(out) -> bus_creator/6  "CoolantFanStepAct"
  OilPressureWarning/1(out) -> bus_creator/7  "OilPressureWarning"
  EngIdlShutDwnTxt_D_Rq/1(out) -> bus_creator/8  "EngIdlShutDwnTxt_D_Rq"
  TrnTotLss_Tq_Est/1(out) -> bus_creator/9  "TrnTotLss_Tq_Est"
  TrnTotTq_Rt_Est/1(out) -> bus_creator/10  "TrnTotTq_Rt_Est"
  AirCondFluidHi_P_Actl/1(out) -> bus_creator/11  "AirCondFluidHi_P_Actl"
  FUEL_ALCOHOL_PERCNT/1(out) -> bus_creator/12  "FUEL_ALCOHOL_PERCNT"
  bus_selector/1 -> VehVLimActv_B_Actl/1(in)  "<VehVLimActv_B_Actl>"
  bus_selector/2 -> VehVLimStat_D_Actl/1(in)  "<VehVLimStat_D_Actl>"
  bus_selector/3 -> ECMMILRequest/1(in)  "<ECMMILRequest>"
  bus_selector/4 -> FohEng_D_Rq/1(in)  "<FohEng_D_Rq>"
  bus_selector/5 -> EngIdlShutDown_D_Stat/1(in)  "<EngIdlShutDown_D_Stat>"
  bus_selector/6 -> CoolantFanStepAct/1(in)  "<CoolantFanStepAct>"
  bus_selector/7 -> OilPressureWarning/1(in)  "<OilPressureWarning>"
  bus_selector/8 -> EngIdlShutDwnTxt_D_Rq/1(in)  "<EngIdlShutDwnTxt_D_Rq>"
  bus_selector/9 -> TrnTotLss_Tq_Est/1(in)  "<TrnTotLss_Tq_Est>"
  bus_selector/10 -> TrnTotTq_Rt_Est/1(in)  "<TrnTotTq_Rt_Est>"
  bus_selector/11 -> AirCondFluidHi_P_Actl/1(in)  "<AirCondFluidHi_P_Actl>"
  bus_selector/12 -> FUEL_ALCOHOL_PERCNT/1(in)  "<FUEL_ALCOHOL_PERCNT>"
  in/1 -> bus_selector/1

== system test_mdl_NI/CAN_Signal/ECM_DIESEL PCM PCM_HEV/PowertrainData_2_0x42D ==
  in : Inport
  ApedPos_Pc_ActlDiag : Subsystem
  EngAirIn_Te_Actl : Subsystem
  EngClnt_Te_ActlDiag : Subsystem
  EngLoad_Pc_CalcDiag : Subsystem
  EngMsgTxt_D_Rq : Subsystem
  GrllShtrPos_B_Falt : Subsystem
  GrllShtrPos_D_Cmd : Subsystem
  IsaOffst_D_Stat : Subsystem
  ObdWarmUp_B_Complt : Subsystem
  SlMde_D_RqDsply : Subsystem
  SlMde_D_Stat : Subsystem
  bus_creator : BusCreator  Inputs=11
  bus_selector : BusSelector  OutputSignals=ObdWarmUp_B_Complt,EngMsgTxt_D_Rq,EngAirIn_Te_Actl,ApedPos_Pc_ActlDiag,EngClnt_Te_ActlDiag,EngLoad_Pc_CalcDiag,GrllShtrPos_D_Cmd,GrllShtrPos_B_Falt,IsaOffst_D_Stat,SlMde_D_RqDsply,SlMde_D_Stat
  out_port : Outport
  wires:
  bus_creator/1 -> out_port/1  "PowertrainData_2_0x42D"
  ObdWarmUp_B_Complt/1(out) -> bus_creator/1  "ObdWarmUp_B_Complt"
  EngMsgTxt_D_Rq/1(out) -> bus_creator/2  "EngMsgTxt_D_Rq"
  EngAirIn_Te_Actl/1(out) -> bus_creator/3  "EngAirIn_Te_Actl"
  ApedPos_Pc_ActlDiag/1(out) -> bus_creator/4  "ApedPos_Pc_ActlDiag"
  EngClnt_Te_ActlDiag/1(out) -> bus_creator/5  "EngClnt_Te_ActlDiag"
  EngLoad_Pc_CalcDiag/1(out) -> bus_creator/6  "EngLoad_Pc_CalcDiag"
  GrllShtrPos_D_Cmd/1(out) -> bus_creator/7  "GrllShtrPos_D_Cmd"
  GrllShtrPos_B_Falt/1(out) -> bus_creator/8  "GrllShtrPos_B_Falt"
  IsaOffst_D_Stat/1(out) -> bus_creator/9  "IsaOffst_D_Stat"
  SlMde_D_RqDsply/1(out) -> bus_creator/10  "SlMde_D_RqDsply"
  SlMde_D_Stat/1(out) -> bus_creator/11  "SlMde_D_Stat"
  bus_selector/1 -> ObdWarmUp_B_Complt/1(in)  "<ObdWarmUp_B_Complt>"
  bus_selector/2 -> EngMsgTxt_D_Rq/1(in)  "<EngMsgTxt_D_Rq>"
  bus_selector/3 -> EngAirIn_Te_Actl/1(in)  "<EngAirIn_Te_Actl>"
  bus_selector/4 -> ApedPos_Pc_ActlDiag/1(in)  "<ApedPos_Pc_ActlDiag>"
  bus_selector/5 -> EngClnt_Te_ActlDiag/1(in)  "<EngClnt_Te_ActlDiag>"
  bus_selector/6 -> EngLoad_Pc_CalcDiag/1(in)  "<EngLoad_Pc_CalcDiag>"
  bus_selector/7 -> GrllShtrPos_D_Cmd/1(in)  "<GrllShtrPos_D_Cmd>"
  bus_selector/8 -> GrllShtrPos_B_Falt/1(in)  "<GrllShtrPos_B_Falt>"
  bus_selector/9 -> IsaOffst_D_Stat/1(in)  "<IsaOffst_D_Stat>"
  bus_selector/10 -> SlMde_D_RqDsply/1(in)  "<SlMde_D_RqDsply>"
  bus_selector/11 -> SlMde_D_Stat/1(in)  "<SlMde_D_Stat>"
  in/1 -> bus_selector/1

== system test_mdl_NI/CAN_Signal/ECM_DIESEL PCM PCM_HEV/PowertrainData_3_0x43E ==
  in : Inport
  BattULoChrg_U_Cmd : Subsystem
  ElLoadCtl_D_Rq : Subsystem
  EngMnfld_P_Actl : Subsystem
  FuelPumpPwr_B_Rq : Subsystem
  bus_creator : BusCreator  Inputs=4
  bus_selector : BusSelector  OutputSignals=BattULoChrg_U_Cmd,ElLoadCtl_D_Rq,FuelPumpPwr_B_Rq,EngMnfld_P_Actl
  out_port : Outport
  wires:
  bus_creator/1 -> out_port/1  "PowertrainData_3_0x43E"
  BattULoChrg_U_Cmd/1(out) -> bus_creator/1  "BattULoChrg_U_Cmd"
  ElLoadCtl_D_Rq/1(out) -> bus_creator/2  "ElLoadCtl_D_Rq"
  FuelPumpPwr_B_Rq/1(out) -> bus_creator/3  "FuelPumpPwr_B_Rq"
  EngMnfld_P_Actl/1(out) -> bus_creator/4  "EngMnfld_P_Actl"
  bus_selector/1 -> BattULoChrg_U_Cmd/1(in)  "<BattULoChrg_U_Cmd>"
  bus_selector/2 -> ElLoadCtl_D_Rq/1(in)  "<ElLoadCtl_D_Rq>"
  bus_selector/3 -> FuelPumpPwr_B_Rq/1(in)  "<FuelPumpPwr_B_Rq>"
  bus_selector/4 -> EngMnfld_P_Actl/1(in)  "<EngMnfld_P_Actl>"
  in/1 -> bus_selector/1

== system test_mdl_NI/CAN_Signal/ECM_DIESEL PCM PCM_HEV/PowertrainData_6_0x205 ==
  in : Inport
  BrkTot_Tq_RqFapLc : Subsystem
  FapLc_B_Err : Subsystem
  TrnAin_Pc_RqDrv : Subsystem
  bus_creator : BusCreator  Inputs=3
  bus_selector : BusSelector  OutputSignals=BrkTot_Tq_RqFapLc,FapLc_B_Err,TrnAin_Pc_RqDrv
  out_port : Outport
  wires:
  bus_creator/1 -> out_port/1  "PowertrainData_6_0x205"
  BrkTot_Tq_RqFapLc/1(out) -> bus_creator/1  "BrkTot_Tq_RqFapLc"
  FapLc_B_Err/1(out) -> bus_creator/2  "FapLc_B_Err"
  TrnAin_Pc_RqDrv/1(out) -> bus_creator/3  "TrnAin_Pc_RqDrv"
  bus_selector/1 -> BrkTot_Tq_RqFapLc/1(in)  "<BrkTot_Tq_RqFapLc>"
  bus_selector/2 -> FapLc_B_Err/1(in)  "<FapLc_B_Err>"
  bus_selector/3 -> TrnAin_Pc_RqDrv/1(in)  "<TrnAin_Pc_RqDrv>"
  in/1 -> bus_selector/1

== system test_mdl_NI/CAN_Signal/ECM_DIESEL PCM PCM_HEV/PowertrainData_7_0x41F ==
  in : Inport
  EcoCochA_Pc_Dsply : Subsystem
  EcoCochCrus_Pc_Dsply : Subsystem
  EcoCochDecel_Pc_Dsply : Subsystem
  EcoCochIdlFuel_Pc_Dsply : Subsystem
  EcoCochInstNeg_B_Dsply : Subsystem
  EcoCochInst_Pc_Dsply : Subsystem
  EcoCochShif_Pc_Dsply : Subsystem
  bus_creator : BusCreator  Inputs=7
  bus_selector : BusSelector  OutputSignals=EcoCochA_Pc_Dsply,EcoCochCrus_Pc_Dsply,EcoCochDecel_Pc_Dsply,EcoCochIdlFuel_Pc_Dsply,EcoCochShif_Pc_Dsply,EcoCochInst_Pc_Dsply,EcoCochInstNeg_B_Dsply
  out_port : Outport
  wires:
  bus_creator/1 -> out_port/1  "PowertrainData_7_0x41F"
  EcoCochA_Pc_Dsply/1(out) -> bus_creator/1  "EcoCochA_Pc_Dsply"
  EcoCochCrus_Pc_Dsply/1(out) -> bus_creator/2  "EcoCochCrus_Pc_Dsply"
  EcoCochDecel_Pc_Dsply/1(out) -> bus_creator/3  "EcoCochDecel_Pc_Dsply"
  EcoCochIdlFuel_Pc_Dsply/1(out) -> bus_creator/4  "EcoCochIdlFuel_Pc_Dsply"
  EcoCochShif_Pc_Dsply/1(out) -> bus_creator/5  "EcoCochShif_Pc_Dsply"
  EcoCochInst_Pc_Dsply/1(out) -> bus_creator/6  "EcoCochInst_Pc_Dsply"
  EcoCochInstNeg_B_Dsply/1(out) -> bus_creator/7  "EcoCochInstNeg_B_Dsply"
  bus_selector/1 -> EcoCochA_Pc_Dsply/1(in)  "<EcoCochA_Pc_Dsply>"
  bus_selector/2 -> EcoCochCrus_Pc_Dsply/1(in)  "<EcoCochCrus_Pc_Dsply>"
  bus_selector/3 -> EcoCochDecel_Pc_Dsply/1(in)  "<EcoCochDecel_Pc_Dsply>"
  bus_selector/4 -> EcoCochIdlFuel_Pc_Dsply/1(in)  "<EcoCochIdlFuel_Pc_Dsply>"
  bus_selector/5 -> EcoCochShif_Pc_Dsply/1(in)  "<EcoCochShif_Pc_Dsply>"
  bus_selector/6 -> EcoCochInst_Pc_Dsply/1(in)  "<EcoCochInst_Pc_Dsply>"
  bus_selector/7 -> EcoCochInstNeg_B_Dsply/1(in)  "<EcoCochInstNeg_B_Dsply>"
  in/1 -> bus_selector/1
